simulink model "Multimotor_GuidanceModel_UAV_Animation"  (R2024b)
settings: Solver=VariableStepAuto  StartTime=0.0  StopTime=10.0  RelTol=1e-3
undefined symbols (not defined in the file): Pitch, Roll, Thrust, YawRate
libraries: uavalgslib x1, uavutilslib x1

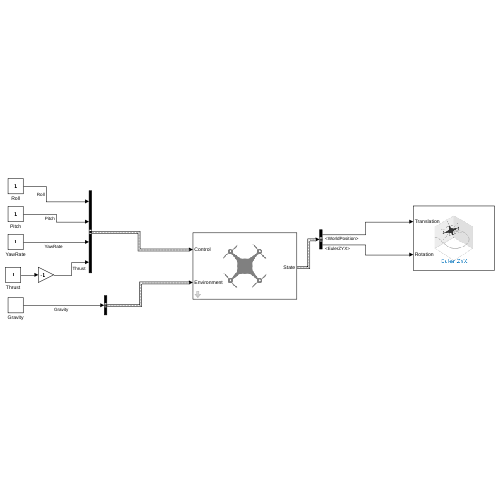
[thumbnail: Simulink's stored preview of the top-level diagram]
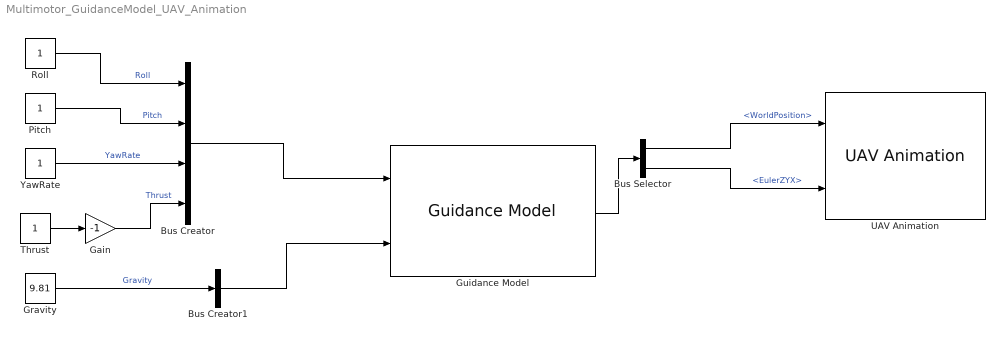
== system Multimotor_GuidanceModel_UAV_Animation ==
  Bus Creator : BusCreator  Inputs=Roll,Pitch,YawRate,Thrust  OutDataTypeStr=Bus: MultirotorGuidanceControlBus  NonVirtualBus=on
  Bus Creator1 : BusCreator  Inputs=Gravity  OutDataTypeStr=Bus: MultirotorGuidanceEnvironmentBus  NonVirtualBus=on
  Bus Selector : BusSelector  OutputSignals=WorldPosition,EulerZYX
  Gain : Gain  Gain=-1
  Gravity : Constant  Value=9.81
  Guidance Model : uavalgslib/Guidance Model  ModelType=MultirotorGuidance  SpecifiedDataType=double  SimulateUsing=Interpreted execution  InitialWorldPositionMultirotor=[0; 0; 0]  InitialWorldVelocityMultirotor=[0; 0; 0]  InitialEulerZYXMultirotor=[0; 0; 0]  InitialBodyAngularRateRPYMultirotor=[0; 0; 0]  InitialThrustMultirotor=0  InitialNorthFixedWing=0  InitialEastFixedWing=0  InitialHeightFixedWing=0  InitialAirSpeedFixedWing=0  InitialHeadingAngleFixedWing=0  InitialFlightPathAngleFixedWing=0  InitialRollAngleFixedWing=0  InitialRollAngleRateFixedWing=0  PDRollMultirotor=[3402.97,116.67]  PDPitchMultirotor=[3402.97, 116.67]  PYawRateMultirotor=1950  PThrustMultirotor=3900  MassMultirotor=0.1  PHeightFixedWing=3.9  PHeadingAngleFixedWing=3.9  PFlightPathAngleFixedWing=39  PDRollFixedWing=[3402.97, 116.67]  PAirSpeedFixedWing=1  FlightPathAngleLimitsFixedWing=[-pi/2, pi/2]  StateBusName='MultirotorGuidanceStateBus'  ControlBusName='MultirotorGuidanceControlBus'  EnvironmentBusName='MultirotorGuidanceEnvironmentBus'  DataType=double
  Pitch : Constant
  Roll : Constant
  Thrust : Constant
  UAV Animation : uavutilslib/UAV Animation  NumUAV=1  DynamicUAVConfig=off  UAVType=Multirotor  UAVSize=1  UAVColor=[1 0 0]  UAVTrajectoryAlpha=1  InertialZDirection=Down  RotationFormat=Euler ZYX  DrawMarkers=off  SampleTime=-1
  YawRate : Constant
  wires:
  Bus Selector/2 -> UAV Animation/2  "<EulerZYX>"
  Bus Selector/1 -> UAV Animation/1  "<WorldPosition>"
  Bus Creator1/1 -> Guidance Model/2
  Roll/1 -> Bus Creator/1  "Roll"
  Bus Creator/1 -> Guidance Model/1
  YawRate/1 -> Bus Creator/3  "YawRate"
  Guidance Model/1 -> Bus Selector/1
  Gravity/1 -> Bus Creator1/1  "Gravity"
  Pitch/1 -> Bus Creator/2  "Pitch"
  Thrust/1 -> Gain/1
  Gain/1 -> Bus Creator/4  "Thrust"
